simulink model "sistemaUno"  (R2018b)
settings: Solver=ode45  StartTime=0.0  StopTime=48  RelTol=1e-5  EnableMultiTasking=on
values from neighbouring files (symbols this model uses):
  n_inicial = 1    [inicializarVariablesSist1.m]
  s_inicial = 50    [inicializarVariablesSist1.m]
  x_inicial = 1    [inicializarVariablesSist1.m]
settings Model: Creator=juan_  LastModifiedBy=barcala
settings DataIOCC: LimitDataPoints=on  SaveFormat=Array
settings OptimizationCC: LifeSpan=inf
settings DebuggingCC: UnderspecifiedInitializationDetection=Classic  MergeDetectMultiDrivingBlocksExec=none  SolverPrmCheckMsg=warning  SFUnexpectedBacktrackingDiag=warning  SFNoUnconditionalDefaultTransitionDiag=warning  SFExecutionAtInitializationDiag=none
settings HardwareCC: ProdBitPerPointer=32  ProdBitPerSizeT=32  ProdBitPerPtrDiffT=32  ProdLargestAtomicFloat=None  ProdIntDivRoundTo=Undefined  ProdEndianess=Unspecified  ProdWordSize=32  ProdHWDeviceType=32-bit Generic
settings ModelReferenceCC: PropagateSignalLabelsOutOfModel=off
settings SFSimCC: SimUseLocalCustomCode=off
settings RTWCC: RTWUseLocalCustomCode=off
settings CodeAppCC: StateflowObjectComments=on
settings GRTTargetCC: TargetLangStandard=C89/C90 (ANSI)  GeneratePreprocessorConditionals=Disable all
settings ConfigComp: CovMetricSettings=dw  CovHtmlReporting=on  CovSaveCumulativeToWorkspaceVar=on  CovSaveSingleToWorkspaceVar=on  CovExternalEMLEnable=off

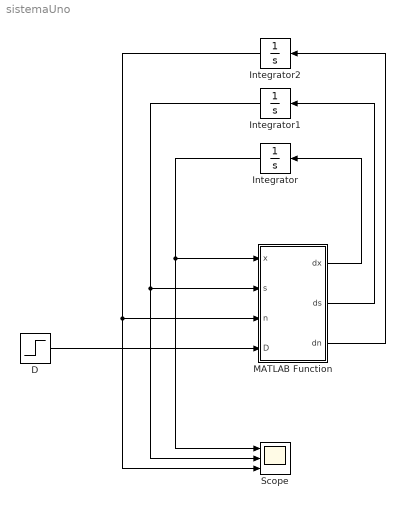
== system sistemaUno ==
  "D " : Step  Time=7  After=0.25  SampleTime=0
  Integrator : Integrator  InitialCondition=x_inicial
  Integrator1 : Integrator  InitialCondition=s_inicial
  Integrator2 : Integrator  InitialCondition=n_inicial
  MATLAB Function : MATLAB Function  TreatAsAtomicUnit=on
  Scope : Scope  NumInputPorts=3
  wires:
  MATLAB Function/1(dx) -> Integrator/1
  Integrator/1 -> MATLAB Function/1(x), Scope/1
  MATLAB Function/2(ds) -> Integrator1/1
  MATLAB Function/3(dn) -> Integrator2/1
  Integrator1/1 -> MATLAB Function/2(s), Scope/2
  Integrator2/1 -> Scope/3, MATLAB Function/3(n)
  "D "/1 -> MATLAB Function/4(D)

== matlab function sistemaUno/MATLAB Function ==
  data: x input; dx output; s input; n input; ds output; dn output; D input
function [dx,ds,dn] = fcn(x,s,n,D)

k1=1/0.45;
k2=0.108;
s_in=50;
n_in=5;

mu_max=0.5;
Ks=0.5;
rx=x*mu_max*s/(Ks+s);
rs=-k1*rx;
rn=-k2*rx;

dx= rx+D*(-x);
ds= rs+D*(s_in-s);
dn= rn+D*(n_in-n);
